simulink model "sampleModel1840_2_sub"  (R2023a)
settings: Solver=VariableStepAuto  StartTime=0.0  StopTime=10.0  RelTol=1e-3
libraries: hdlsllib x6, simulink x2
settings Model: Creator=user1  LastModifiedBy=user1

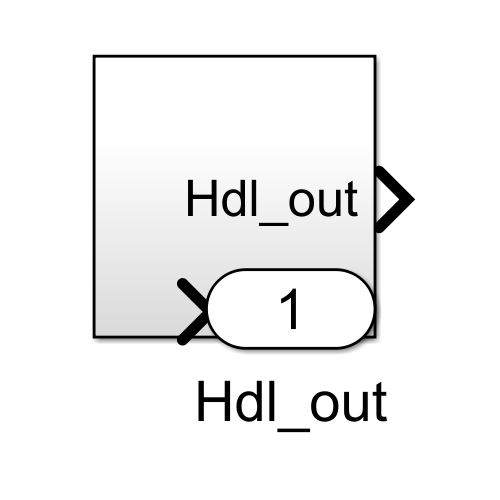
[thumbnail: Simulink's stored preview of the top-level diagram]
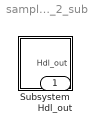
== system sampleModel1840_2_sub ==
  Subsystem : Subsystem
  Hdl_out : Outport  OutDataTypeStr=uint8

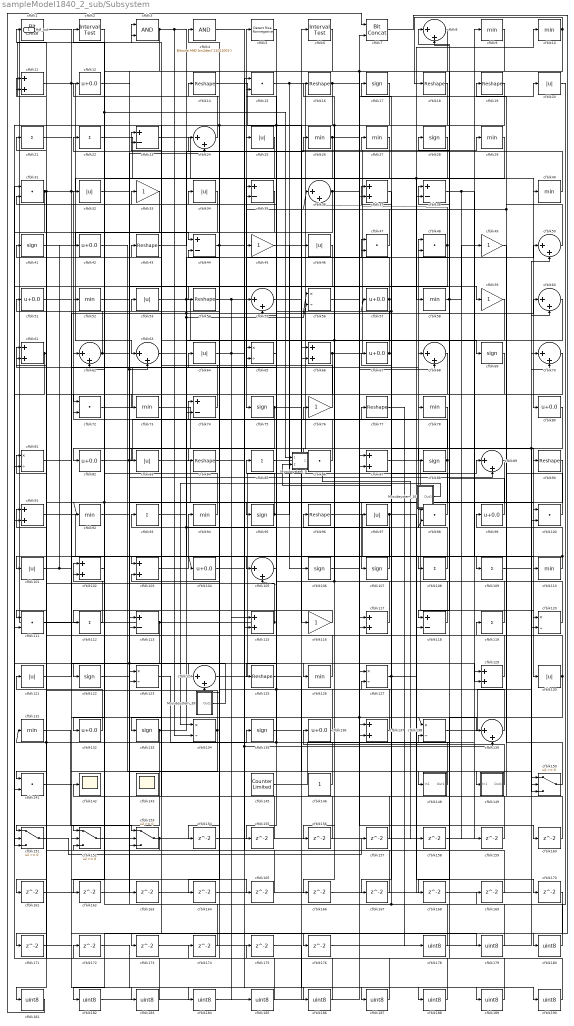
== system sampleModel1840_2_sub/Subsystem ==
  Mysubsystem_16 : Subsystem  TreatAsAtomicUnit=on  RTWFcnName=Mysubsystem_16
      settings: RTWFcnNameOpts=User specified  RTWFileNameOpts=Use function name
  Mysubsystem_39 : Subsystem  TreatAsAtomicUnit=on  RTWFcnName=Mysubsystem_39
      settings: RTWFcnNameOpts=User specified  RTWFileNameOpts=Use function name
  Mysubsystem_9 : Subsystem  TreatAsAtomicUnit=on  RTWFcnName=Mysubsystem_9
      settings: RTWFcnNameOpts=User specified  RTWFileNameOpts=Use function name
  cfblk1 : simulink/Logic and Bit Operations/Bit Clear  iBit=0
      settings: LibrarySourceBlock=|
      | hdlsllib/Logic and Bit
      | Operations/Bit Clear
  cfblk{9..10,26..27,29,40,52,58,73,78,92,94,110,126,131} (15 alike) : MinMax  OutDataTypeStr=uint8
  cfblk{15,31,47..48,72,86,98,100,111,141} (10 alike) : DotProduct  OutDataTypeStr=uint8
  cfblk{20,25,32,34,46,53,64,83,97,101,121,130} (12 alike) : Abs  OutDataTypeStr=uint8  SaturateOnIntegerOverflow=off
  cfblk{11,37,61,66,87,91,102..103,115,117,129,137} (12 alike) : Sum  OutDataTypeStr=uint8
  cfblk{12,42,51,57,67,80,82,99,104,132,136} (11 alike) : Bias  Bias=0.0  SaturateOnIntegerOverflow=off
  cfblk{8,24,36,50,55,60,62..63,68,70,89,105,124,139} (14 alike) : Sum  Inputs=|++  OutDataTypeStr=uint8
  cfblk{17,28,41,69,75,88,95,106..107,122,133,135} (12 alike) : Signum
  cfblk{21..22,85,93,108..109,112,119} (8 alike) : Sum  Inputs=+  OutDataTypeStr=uint8
  cfblk{23,35,38,44,74,113,118} (7 alike) : Sum  Inputs=+-  OutDataTypeStr=uint8
  cfblk{33,45,49,59,76,116} (6 alike) : Gain  OutDataTypeStr=uint8
  cfblk{56,65,81,120,123,127,134,138} (8 alike) : Product  Inputs=*/  OutDataTypeStr=uint8  RndMeth=Zero  SaturateOnIntegerOverflow=on
  cfblk{14,16,18..19,43,54,77,84,90,96,125} (11 alike) : Reshape
  cfblk142 : Scope
  cfblk143 : Scope
      settings: Floating=on
  cfblk145 : hdlsllib/Sources/Counter Limited  uplimit=7  tsamp=-1
  cfblk146 : Constant  OutDataTypeStr=uint8  SampleTime=-1
  cfblk148 : Subsystem
      settings: LibrarySourceBlock=|
      | hdlsllib/Ports &
      | Subsystems/Subsystem
  cfblk149 : Subsystem
      settings: LibrarySourceBlock=|
      | hdlsllib/Ports &
      | Subsystems/Subsystem
  cfblk{150..153} (4 alike) : Switch  OutDataTypeStr=uint8  SaturateOnIntegerOverflow=off  InputSameDT=off
  cfblk{154..176} (23 alike) : Delay  SampleTime=1
  cfblk{178..190} (13 alike) : DataTypeConversion  OutDataTypeStr=uint8  SaturateOnIntegerOverflow=off  RndMeth=Floor
  cfblk2 : hdlsllib/Logic and Bit Operations/Interval Test  IntervalClosedRight=on  uplimit=0.5  IntervalClosedLeft=on  lowlimit=-0.5  OutDataTypeStr=uint8
  cfblk3 : Logic  AllPortsSameDT=off  OutDataTypeStr=boolean
  cfblk4 : simulink/Logic and Bit Operations/Bitwise Operator  logicop=AND  UseBitMask=on  BitMask=bin2dec('11011001')  BitMaskRealWorld=Stored Integer
      settings: LibrarySourceBlock=|
      | hdlsllib/Logic and Bit
      | Operations/Bitwise
      | Operator
  cfblk5 : hdlsllib/Logic and Bit Operations/Detect Rise Nonnegative  vinit=0  OutDataTypeStr=uint8
  cfblk6 : hdlsllib/Logic and Bit Operations/Interval Test  IntervalClosedRight=on  uplimit=0.5  IntervalClosedLeft=on  lowlimit=-0.5  OutDataTypeStr=uint8
  cfblk7 : hdlsllib/Logic and Bit Operations/Bit Concat  numInputs=2
  Hdl_out : Outport  OutDataTypeStr=uint8
  wires:
  cfblk42/1 -> cfblk149/1(In1)
  cfblk112/1 -> cfblk102/1
  cfblk54/1 -> cfblk190/1, cfblk185/1
  cfblk123/1 -> cfblk135/1
  cfblk49/1 -> cfblk142/1
  cfblk139/1 -> cfblk33/1
  cfblk108/1 -> cfblk48/1
  cfblk103/1 -> cfblk94/1
  cfblk117/1 -> cfblk16/1, cfblk93/1
  cfblk124/1 -> cfblk89/1
  cfblk120/1 -> cfblk34/1
  cfblk22/1 -> cfblk58/1
  cfblk59/1 -> cfblk156/1, cfblk103/1
  cfblk11/1 -> cfblk139/1, cfblk63/1
  cfblk132/1 -> cfblk121/1
  cfblk66/1 -> cfblk153/3, cfblk29/1
  cfblk133/1 -> cfblk171/1, cfblk98/2, cfblk78/1
  cfblk82/1 -> cfblk68/1, cfblk74/1
  cfblk131/1 -> cfblk153/1
  cfblk62/1 -> cfblk21/1, cfblk86/1
  cfblk25/1 -> cfblk92/1, cfblk122/1
  cfblk12/1 -> cfblk89/2
  cfblk72/1 -> cfblk5/1
  cfblk121/1 -> cfblk64/1
  cfblk15/1 -> cfblk106/1, cfblk130/1
  cfblk91/1 -> cfblk127/1
  cfblk61/1 -> cfblk151/3, cfblk3/1
  cfblk23/1 -> cfblk80/1
  cfblk118/1 -> cfblk61/1
  cfblk95/1 -> cfblk46/1, cfblk85/1
  cfblk136/1 -> cfblk15/2, cfblk51/1
  cfblk83/1 -> cfblk117/2
  cfblk32/1 -> cfblk59/1
  cfblk57/1 -> cfblk164/1, cfblk25/1
  cfblk134/1 -> cfblk152/2, cfblk81/1
  cfblk84/1 -> cfblk126/1
  cfblk31/1 -> cfblk141/2, cfblk141/1, cfblk40/1, cfblk137/2, cfblk138/1
  cfblk90/1 -> cfblk107/1
  cfblk87/1 -> cfblk120/1
  cfblk63/1 -> cfblk56/2, cfblk47/1
  cfblk85/1 -> cfblk50/1
  cfblk116/1 -> cfblk112/1
  cfblk64/1 -> cfblk115/1, cfblk176/1, cfblk139/2
  cfblk75/1 -> cfblk90/1, cfblk82/1
  cfblk119/1 -> cfblk67/1
  cfblk67/1 -> cfblk35/2, Mysubsystem_9/2(In2)
  cfblk146/1 -> cfblk11/2, cfblk131/1
  cfblk36/1 -> cfblk91/2, cfblk137/1
  cfblk149/1(Out1) -> cfblk136/1
  cfblk150/1 -> cfblk22/1
  cfblk99/1 -> cfblk8/1
  cfblk34/1 -> cfblk73/1
  cfblk50/1 -> cfblk23/1
  cfblk41/1 -> cfblk44/1
  cfblk55/1 -> cfblk116/1
  cfblk70/1 -> cfblk84/1
  cfblk77/1 -> cfblk178/1
  cfblk153/1 -> cfblk152/3, cfblk129/1
  cfblk94/1 -> cfblk2/1
  cfblk27/1 -> cfblk75/1
  cfblk76/1 -> cfblk41/1
  cfblk26/1 -> cfblk68/2, cfblk83/1
  cfblk38/1 -> cfblk159/1, cfblk110/1
  cfblk46/1 -> cfblk81/2
  cfblk10/1 -> cfblk98/1, cfblk18/1
  cfblk127/1 -> cfblk10/1, cfblk57/1, cfblk17/1
  cfblk3/1 -> cfblk113/2, cfblk134/2, cfblk105/1
  cfblk43/1 -> cfblk26/1
  cfblk24/1 -> cfblk12/1
  cfblk73/1 -> cfblk150/1
  cfblk138/1 -> cfblk70/2
  cfblk16/1 -> cfblk115/2, cfblk150/2
  cfblk148/1(Out1) -> cfblk105/2, cfblk53/1
  cfblk81/1 -> cfblk60/1
  cfblk96/1 -> cfblk108/1
  cfblk106/1 -> cfblk20/1
  cfblk40/1 -> cfblk24/1
  cfblk53/1 -> cfblk69/1, cfblk87/1
  cfblk45/1 -> cfblk120/2
  cfblk89/1 -> cfblk151/1
  cfblk107/1 -> cfblk96/1
  cfblk74/1 -> cfblk31/2
  cfblk21/1 -> cfblk109/1
  cfblk29/1 -> cfblk95/1
  cfblk88/1 -> cfblk124/2, cfblk32/1
  cfblk93/1 -> cfblk47/2, cfblk56/1
  cfblk19/1 -> cfblk133/1, cfblk124/1
  cfblk8/1 -> cfblk152/1, Mysubsystem_9/1(In1)
  cfblk104/1 -> cfblk76/1
  cfblk137/1 -> cfblk103/2
  cfblk44/1 -> cfblk154/1, cfblk88/1
  cfblk97/1 -> cfblk170/1, cfblk101/1
  cfblk80/1 -> cfblk118/1, cfblk150/3
  cfblk6/1 -> cfblk55/2
  cfblk135/1 -> cfblk27/1
  cfblk100/1 -> cfblk19/1, cfblk36/1
  cfblk98/1 -> cfblk37/1
  cfblk113/1 -> cfblk132/1, cfblk43/1
  cfblk28/1 -> cfblk38/2, cfblk123/2
  cfblk122/1 -> cfblk63/2, cfblk65/1
  cfblk125/1 -> cfblk148/1(In1)
  cfblk2/1 -> cfblk72/1
  cfblk102/1 -> cfblk62/1
  cfblk130/1 -> cfblk168/1, cfblk119/1
  cfblk52/1 -> cfblk100/1
  cfblk65/1 -> cfblk45/1
  cfblk60/1 -> cfblk87/2
  cfblk69/1 -> cfblk111/1
  cfblk109/1 -> cfblk60/2
  cfblk101/1 -> cfblk42/1, cfblk129/2
  cfblk145/1 -> cfblk9/1
  cfblk48/1 -> cfblk54/1, cfblk36/2
  cfblk129/1 -> cfblk91/1
  cfblk115/1 -> Hdl_out/1, cfblk11/1
  cfblk110/1 -> cfblk99/1, cfblk104/1
  cfblk58/1 -> cfblk49/1, cfblk38/1
  cfblk152/1 -> cfblk24/2
  cfblk78/1 -> cfblk97/1
  cfblk105/1 -> cfblk65/2
  cfblk9/1 -> cfblk37/2, cfblk74/2
  cfblk86/1 -> cfblk14/1
  cfblk18/1 -> cfblk166/1, cfblk111/2, cfblk125/1
  cfblk126/1 -> cfblk52/1
  cfblk14/1 -> cfblk66/2
  cfblk47/1 -> cfblk35/1
  cfblk154/1 -> cfblk55/1
  cfblk5/1 -> cfblk155/1
  cfblk155/1 -> cfblk102/2
  cfblk156/1 -> cfblk62/2
  cfblk151/1 -> cfblk157/1
  cfblk157/1 -> cfblk44/2
  cfblk158/1 -> cfblk8/2
  cfblk159/1 -> cfblk23/2
  cfblk56/1 -> cfblk160/1
  cfblk160/1 -> cfblk3/2
  cfblk35/1 -> cfblk161/1
  cfblk161/1 -> cfblk117/1
  cfblk17/1 -> cfblk162/1
  cfblk162/1 -> cfblk66/1
  cfblk92/1 -> cfblk163/1
  cfblk163/1 -> cfblk70/1
  cfblk164/1 -> cfblk118/2
  cfblk111/1 -> cfblk165/1
  cfblk165/1 -> cfblk61/2
  cfblk166/1 -> cfblk100/2
  cfblk37/1 -> cfblk167/1
  cfblk167/1 -> cfblk113/1
  cfblk168/1 -> cfblk138/2
  cfblk20/1 -> cfblk169/1
  cfblk169/1 -> cfblk15/1
  cfblk68/1 -> cfblk173/1
  cfblk173/1 -> cfblk86/2
  cfblk174/1 -> cfblk123/1
  cfblk176/1 -> cfblk50/2
  cfblk178/1 -> cfblk127/2, cfblk72/2
  cfblk51/1 -> cfblk179/1
  cfblk179/1 -> cfblk77/1
  cfblk7/1 -> cfblk180/1
  cfblk180/1 -> cfblk28/1
  cfblk33/1 -> cfblk181/1
  cfblk181/1 -> cfblk7/1
  cfblk170/1 -> cfblk182/1
  cfblk182/1 -> cfblk7/2
  cfblk171/1 -> cfblk183/1
  cfblk183/1 -> cfblk1/1
  cfblk1/1 -> cfblk184/1
  cfblk184/1 -> cfblk6/1
  cfblk185/1 -> cfblk4/1
  cfblk4/1 -> cfblk186/1
  cfblk186/1 -> cfblk174/1
  cfblk172/1 -> cfblk187/1
  cfblk187/1 -> cfblk31/1
  cfblk141/1 -> cfblk188/1
  cfblk188/1 -> cfblk172/1
  cfblk175/1 -> cfblk189/1
  cfblk189/1 -> cfblk48/2
  cfblk190/1 -> cfblk175/1
  Mysubsystem_9/1(Out1) -> cfblk158/1
  Mysubsystem_16/1(Out1) -> cfblk134/1
  Mysubsystem_39/1(Out1) -> cfblk151/2, cfblk153/2

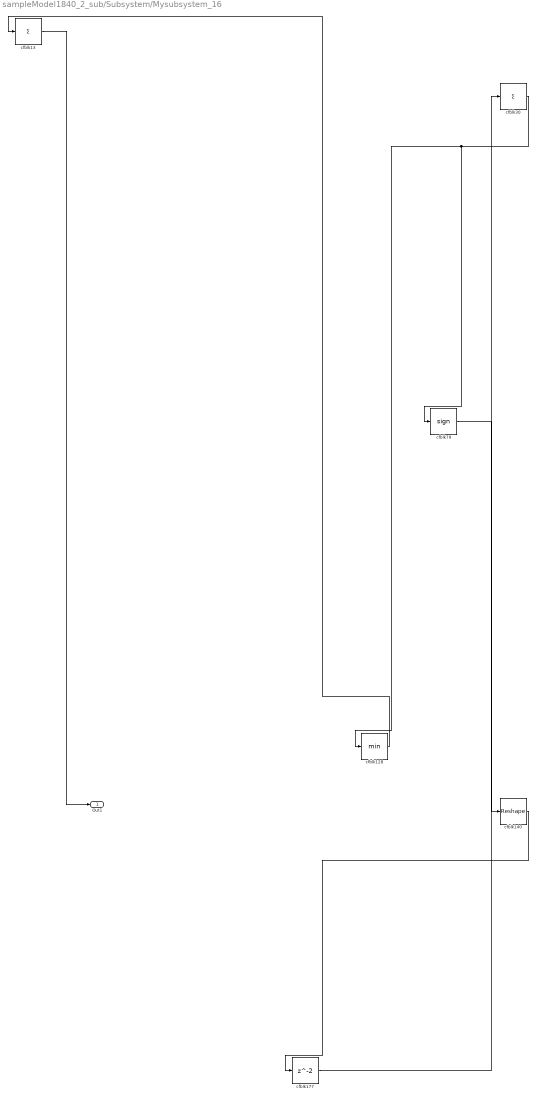
== system sampleModel1840_2_sub/Subsystem/Mysubsystem_16 ==
  cfblk128 : MinMax
  cfblk13 : Sum  Inputs=+
  cfblk140 : Reshape
  cfblk177 : Delay  SampleTime=1
  cfblk30 : Sum  Inputs=+
  cfblk79 : Signum
  Out1 : Outport
  wires:
  cfblk128/1 -> cfblk13/1
  cfblk177/1 -> cfblk30/1
  cfblk30/1 -> cfblk79/1, cfblk128/1
  cfblk140/1 -> cfblk177/1
  cfblk79/1 -> cfblk140/1
  cfblk13/1 -> Out1/1

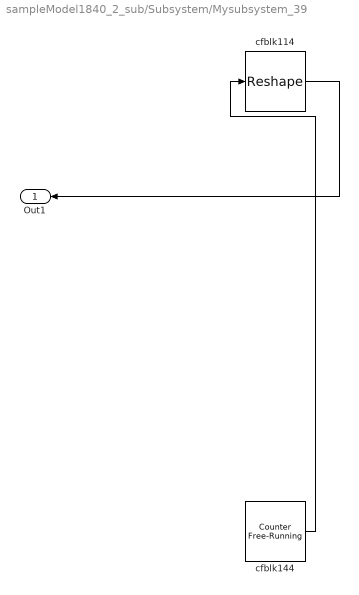
== system sampleModel1840_2_sub/Subsystem/Mysubsystem_39 ==
  cfblk114 : Reshape
  cfblk144 : hdlsllib/Sources/Counter Free-Running  NumBits=16  tsamp=-1
  Out1 : Outport
  wires:
  cfblk114/1 -> Out1/1
  cfblk144/1 -> cfblk114/1

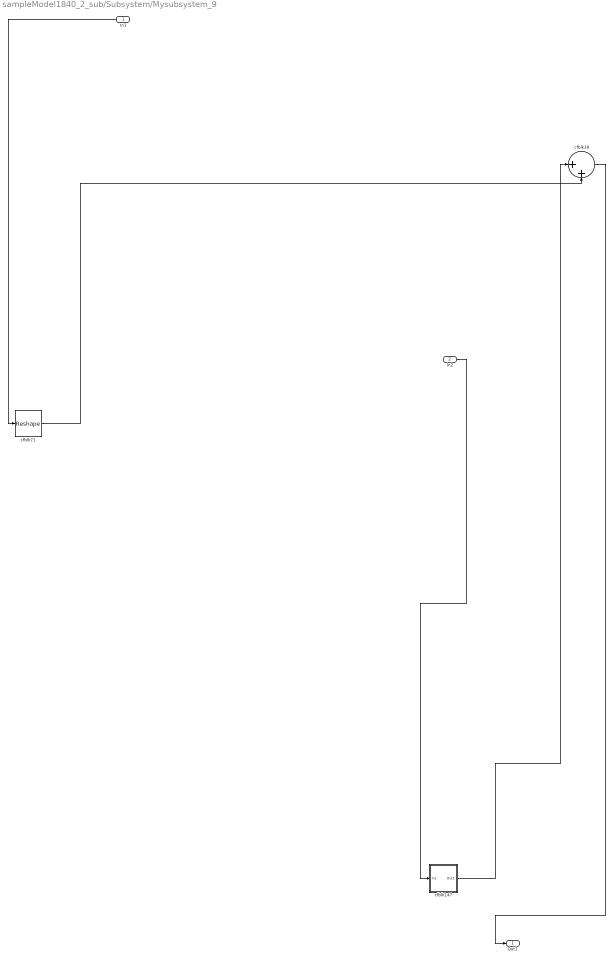
== system sampleModel1840_2_sub/Subsystem/Mysubsystem_9 ==
  In1 : Inport
  In2 : Inport  Port=2
  cfblk147 : Subsystem
      settings: LibrarySourceBlock=|
      | hdlsllib/Ports &
      | Subsystems/Subsystem
  cfblk39 : Sum  Inputs=|++
  cfblk71 : Reshape
  Out1 : Outport
  wires:
  cfblk147/1(Out1) -> cfblk39/1
  cfblk39/1 -> Out1/1
  In1/1 -> cfblk71/1
  In2/1 -> cfblk147/1(In1)
  cfblk71/1 -> cfblk39/2

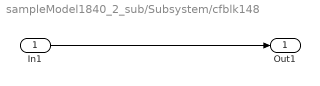
== system sampleModel1840_2_sub/Subsystem/cfblk148 ==
  In1 : Inport
  Out1 : Outport
  wires:
  In1/1 -> Out1/1

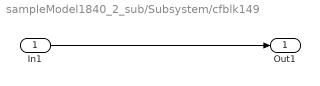
== system sampleModel1840_2_sub/Subsystem/cfblk149 ==
  In1 : Inport
  Out1 : Outport
  wires:
  In1/1 -> Out1/1

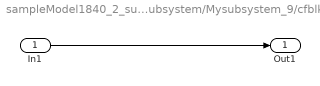
== system sampleModel1840_2_sub/Subsystem/Mysubsystem_9/cfblk147 ==
  In1 : Inport
  Out1 : Outport
  wires:
  In1/1 -> Out1/1
